simulink model "Q2_4"  (R2023b)
settings: Solver=VariableStepAuto  StartTime=0.0  StopTime=100  RelTol=1e-3
libraries: mpclib x1, slpidlib x1, simulink x1
settings Model: Creator=sayed  LastModifiedBy=sayed

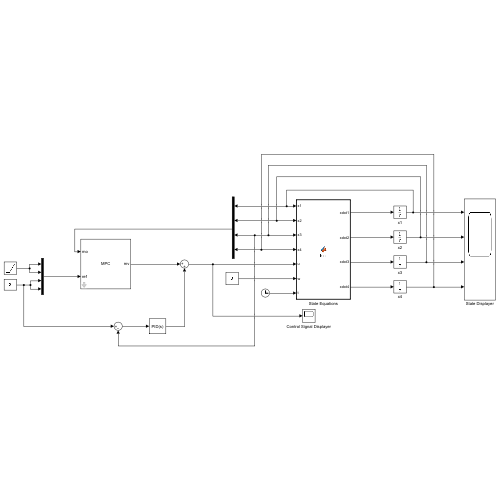
[thumbnail: Simulink's stored preview of the top-level diagram]
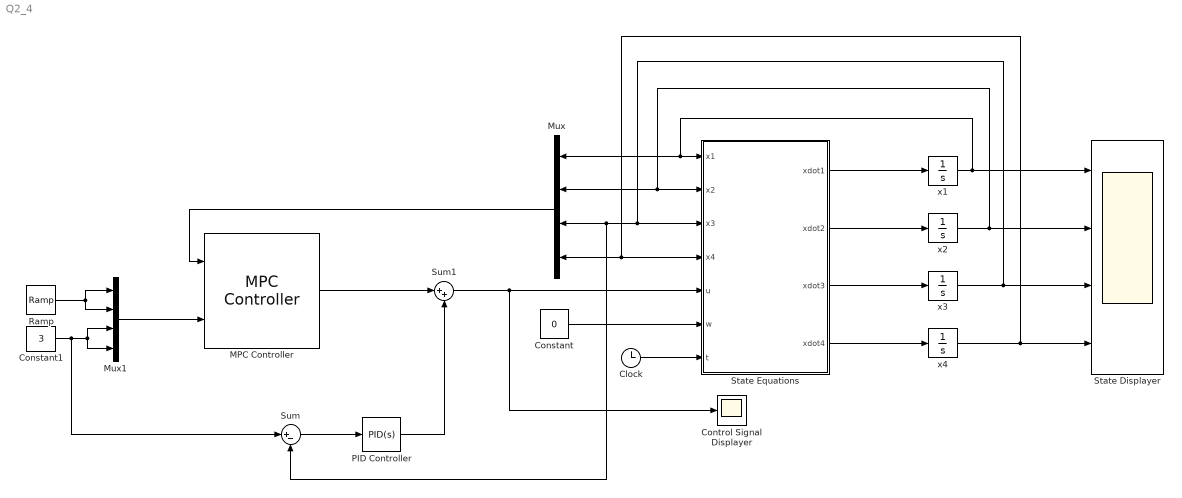
== system Q2_4 ==
  Clock : Clock
  Constant : Constant  Value=0
  Constant1 : Constant  Value=3
  Control Signal Displayer : Scope
  MPC Controller : mpclib/MPC Controller  SCDEnableBlockLinearizationSpecification=on  mpcobj=mpc1  is_multiple=0  enable_value=0  return_u0=off  updateMPCinCallerWorkspace=on  md_inport=off  mv_inport=off  uref_inport=off  return_cost=off  return_mvseq=off  return_qpstatus=off  return_xseq=off  return_state=off  return_ovseq=off  state_inport=off  umin_inport=off  umax_inport=off  ymin_inport=off  ymax_inport=off  cc_inport=off  ywt_inport=off  uwt_inport=off  duwt_inport=off  rhoeps_inport=off  pm_inport=off  MaximumP=10  HorizonChoice=FixedHorizon  n_ts=0.01  n_p=650  n_mv=1  n_md=0  n_ud=0  n_mo=4  n_uo=0  BlockDataType=double  SampleTimeInherited=off  switch_inport=off
  Mux : Mux
  Mux1 : Mux
  PID Controller : slpidlib/PID Controller  Controller=PID  Form=Parallel  TimeDomain=Continuous-time  UseExternalTs=off  SampleTime=-1  IntegratorMethod=Forward Euler  FilterMethod=Forward Euler  ControllerParametersSource=internal  P=1950  I=950  UseKiTs=off  D=0  N=100  UseFilter=on  TunerSelectOption=Transfer Function Based (PID Tuner App)  InitialConditionSource=internal  InitialConditionForIntegrator=0  InitialConditionForFilter=0  DifferentiatorICPrevScaledInput=0  ExternalReset=none  TrackingMode=off  Kt=1  LimitOutput=off  SatLimitsSource=internal  UpperSaturationLimit=inf  LowerSaturationLimit=-inf  LinearizeAsGain=on  AntiWindupMode=none  Kb=1  LimitIntegrator=off  UpperIntegratorSaturationLimit=inf  LowerIntegratorSaturationLimit=-inf  POutMin=[]  POutMax=[]  IOutMin=[]  IOutMax=[]  DOutMin=[]  DOutMax=[]  NOutMin=[]  NOutMax=[]  SumOutMin=[]  SumOutMax=[]  SaturationOutMin=[]  SaturationOutMax=[]  PParamMin=[]  PParamMax=[]  IParamMin=[]  IParamMax=[]  DParamMin=[]  DParamMax=[]  NParamMin=[]  NParamMax=[]  KbParamMin=[]  KbParamMax=[]  KtParamMin=[]  KtParamMax=[]  KbOutMin=[]  KbOutMax=[]  KtOutMin=[]  KtOutMax=[]  IntegratorOutMin=[]  IntegratorOutMax=[]  FilterOutMin=[]  FilterOutMax=[]  SumI1OutMin=[]  SumI1OutMax=[]  SumI2OutMin=[]  SumI2OutMax=[]  SumI3OutMin=[]  SumI3OutMax=[]  SumI4OutMin=[]  SumI4OutMax=[]  SumDOutMin=[]  SumDOutMax=[]  DifferentiatorOutMin=[]  DifferentiatorOutMax=[]  FilterDiffOutCoefMin=[]  FilterDiffOutCoefMax=[]  ReciprocalOutMin=[]  ReciprocalOutMax=[]  SumDenOutMin=[]  SumDenOutMax=[]  SumNumOutMin=[]  SumNumOutMax=[]  DivideOutMin=[]  DivideOutMax=[]  UdiffTsProdOutMin=[]  UdiffTsProdOutMax=[]  NTsProdOutMin=[]  NTsProdOutMax=[]  UintegralTsProdOutMin=[]  UintegralTsProdOutMax=[]  UngainTsProdOutMin=[]  UngainTsProdOutMax=[]  ClampingZeroOutDataTypeStr=Inherit: Inherit via back propagation  ClampingZeroOutMin=[]  ClampingZeroOutMax=[]  FilterDenConstantOutDataTypeStr=Inherit: Inherit via back propagation  FilterDenConstantOutMin=[]  FilterDenConstantOutMax=[]  PCopyOutDataTypeStr=Inherit: Inherit via back propagation  PCopyOutMin=[]  PCopyOutMax=[]  NCopyOutDataTypeStr=Inherit: Inherit via back propagation  NCopyOutMin=[]  NCopyOutMax=[]  IntegratorContinuousStateAttributes=''  IntegratorStateMustResolveToSignalObject=off  IntegratorRTWStateStorageClass=Auto  FilterContinuousStateAttributes=''  FilterStateMustResolveToSignalObject=off  FilterRTWStateStorageClass=Auto  ParallelPVariant=InternalParameters  IdealPVariant=Disabled  IVariant=InternalParameters  DVariant=InternalParameters  IntegratorVariant=Continuous  SatVariant=Disabled  AWVariant=Passthrough  PCopyVariant=Disabled  TRVariant=Disabled  FdbkBlocksVariant=Forward  IdealPFdbkVariant=Disabled  SatFdbkVariant=Disabled  DerivativeFilterVariant=ContFilter  NVariant=InternalParameters  NCopyVariant=Disabled  FilterICVariant=InternalICsFilter  IntegratorICVariant=InternalICs  ExternalResetVariant=Disabled  TRSumVariant=Passthrough  SumFdbkVariant=Disabled  SumVariant=Sum_PID  TsampFilterVariant=InternalTs  TsampNgainVariant=Passthrough  TsampIntegralVariant=Disabled_SignalSpec  ExternalSaturationOutDataTypeStr=Inherit: Same as second input
  Ramp : simulink/Sources/Ramp  slope=3  start=0  InitialOutput=0
  State Displayer : Scope  NumInputPorts=4
  State Equations : MATLAB Function  TreatAsAtomicUnit=on
  Sum : Sum  Inputs=|+-
  Sum1 : Sum  Inputs=|++
  x1 : Integrator
  x2 : Integrator
  x3 : Integrator  InitialCondition=2
  x4 : Integrator  InitialCondition=0.5
  wires:
  State Equations/1(xdot1) -> x1/1
  State Equations/2(xdot2) -> x2/1
  State Equations/3(xdot3) -> x3/1
  State Equations/4(xdot4) -> x4/1
  x1/1 -> State Displayer/1, Mux/1, State Equations/1(x1)
  x2/1 -> State Displayer/2, Mux/2, State Equations/2(x2)
  x3/1 -> State Displayer/3, Mux/3, Sum/2, State Equations/3(x3)
  x4/1 -> State Displayer/4, State Equations/4(x4), Mux/4
  MPC Controller/1 -> Sum1/1
  Ramp/1 -> Mux1/1, Mux1/2
  Mux1/1 -> MPC Controller/2
  Constant1/1 -> Mux1/4, Mux1/3, Sum/1
  Mux/1 -> MPC Controller/1
  Constant/1 -> State Equations/6(w)
  Sum/1 -> PID Controller/1
  Clock/1 -> State Equations/7(t)
  Sum1/1 -> Control Signal Displayer/1, State Equations/5(u)
  PID Controller/1 -> Sum1/2

== matlab function Q2_4/State Equations ==
  data: x1 input; x2 input; x3 input; x4 input; u input; xdot1 output; w input; xdot2 output; xdot3 output; xdot4 output; t input
function [xdot1, xdot2, xdot3, xdot4] = fcn(x1, x2, x3, x4, u, w, t)

% Parameter Values with uncertainity

m1 = 10000;
m1 = m1 + (m1/10) * sin(t);
m2 = 8000;
m2 = m2 + (m2/10) * sin(t);
k = 500000;
k = k + (k/20) * sin(t);
c = 5000;
c = c + (c/20) * sin(t);

% State-Equations

xdot1 = x3;
xdot2 = x4;
xdot3 = (1 / m1) * (k * (-x1 + x2) + c * (-x3 + x4) + u + w);
xdot4 = (1 / m2) * (k * (x1 - x2) + c * (x3 - x4));
